simulink model "planta"  (R2020a)
settings: Solver=VariableStepAuto  StartTime=0.0  StopTime=5  RelTol=1e-3
settings Model: Creator=Sergio  LastModifiedBy=Sergio

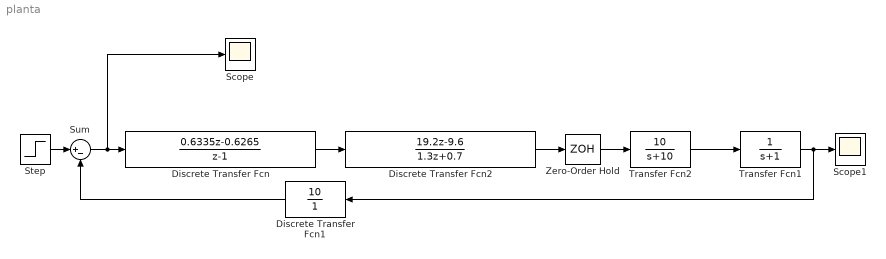
== system planta ==
  Discrete Transfer Fcn : DiscreteTransferFcn  Numerator=[0.6335 -0.6265]  Denominator=[1 -1]
  Discrete Transfer Fcn1 : DiscreteTransferFcn  Numerator=[10]  Denominator=[1]
  Discrete Transfer Fcn2 : DiscreteTransferFcn  Numerator=[19.2 -9.6]  Denominator=[1.3 0.7]
  Scope : Scope
  Scope1 : Scope
  Step : Step  Time=0  SampleTime=0
  Sum : Sum  Inputs=|+-
  Transfer Fcn1 : TransferFcn  Denominator=[1 1]
  Transfer Fcn2 : TransferFcn  Numerator=[10]  Denominator=[1 10]
  Zero-Order Hold : ZeroOrderHold  SampleTime=0.02
  wires:
  Sum/1 -> Scope/1, Discrete Transfer Fcn/1
  Transfer Fcn1/1 -> Discrete Transfer Fcn1/1, Scope1/1
  Discrete Transfer Fcn1/1 -> Sum/2
  Step/1 -> Sum/1
  Zero-Order Hold/1 -> Transfer Fcn2/1
  Transfer Fcn2/1 -> Transfer Fcn1/1
  Discrete Transfer Fcn/1 -> Discrete Transfer Fcn2/1
  Discrete Transfer Fcn2/1 -> Zero-Order Hold/1
